simulink subsystem "altitude_controller"  (R2020a)
settings: Solver=VariableStepAuto  StartTime=0.0  StopTime=10.0  RelTol=1e-3
values from neighbouring files (symbols this model uses):
  balloon_fill_mass = max([      gas_for_equilibrium_at_target, ... (first row only)    [configure_simulation.m]    (also in test_kalman.m = 1.8812)
  combined_dry_mass = payload_dry_mass+m_balloon    [configure_simulation.m]
  consumable_mass = 0.5    [configure_simulation.m]    (also in test_kalman.m = 1)
  delay_altitude = target_altitude-5000    (= 19000)    [configure_simulation.m]
  delay_time = 500    [configure_simulation.m]
  dt = 0.01    [configure_simulation.m]    (also in test_kalman.m)
  max_deadzone_error = 100    [configure_simulation.m]
  max_deadzone_speed = 0.2    [configure_simulation.m]
  mdot_ballast = 0.010    (= 0.01)    [configure_simulation.m]
  mdot_ballast_noise_power = 0.0001    [configure_simulation.m]
  mdot_bleed = 0.010    (= 0.01)    [configure_simulation.m]
  mdot_bleed_noise_power = 0.0001    [configure_simulation.m]
  min_altitude_limit = 15000    [configure_simulation.m]
  target_altitude = 24000    [configure_simulation.m]    (also in linearization.m)
undefined symbols (not defined in the file or in its folder): Dump, enum_ControlMode, max_safe_error, Vent
libraries: simulink x6
settings Model: Creator=Philip  LastModifiedBy=Philip

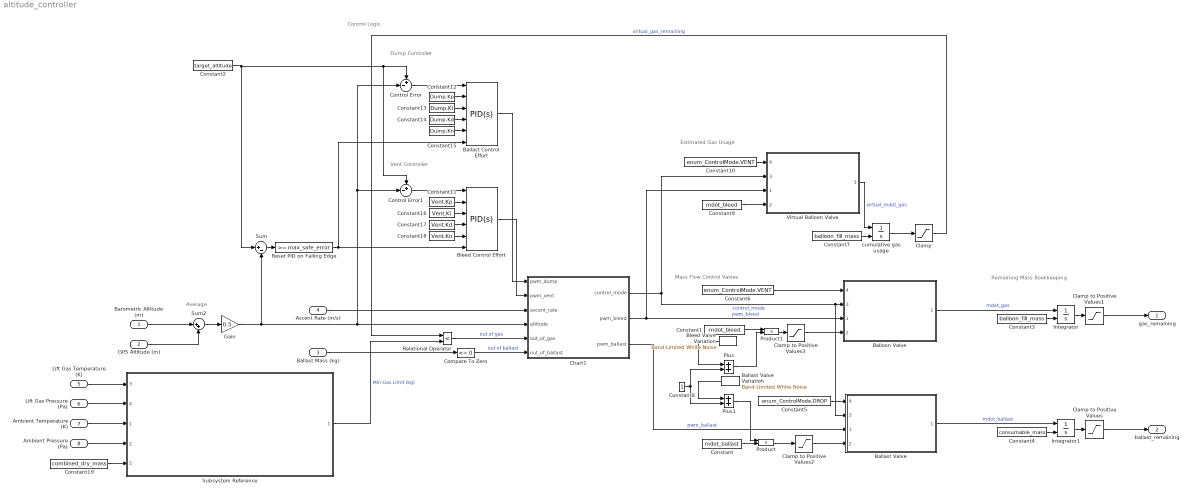
== system altitude_controller ==
  note: Average
  note: Estimated Gas Usage
  note: Remaining Mass Bookkeeping
  note: Mass Flow Control Valves
  note: Control Logic
  note: Dump Controller
  note: Vent Controller
  Barometric Altitude (m) : Inport  Unit=m
  GPS Altitude (m) : Inport  Port=2  OutMin=0  Unit=m
  Ballast Mass (kg) : Inport  Port=3  Unit=kg
  Ascent Rate (m/s) : Inport  Port=4
  Lift Gas Temperature (K) : Inport  Port=5
  Lift Gas Pressure (Pa) : Inport  Port=6
  Ambient Temperature (K) : Inport  Port=7
  Ambient Pressure (Pa) : Inport  Port=8
  Ballast Control Effort : simulink/Continuous/PID Controller  Controller=PID  Form=Parallel  TimeDomain=Continuous-time  UseExternalTs=off  SampleTime=1  IntegratorMethod=Forward Euler  FilterMethod=Forward Euler  ControllerParametersSource=external  P=1  I=1  D=0  UseFilter=on  N=100  TunerSelectOption=Transfer Function Based (PID Tuner App)  InitialConditionSource=internal  InitialConditionForIntegrator=0  InitialConditionForFilter=0  DifferentiatorICPrevScaledInput=0  ExternalReset=falling  TrackingMode=off  Kt=1  LimitOutput=on  UpperSaturationLimit=1  LowerSaturationLimit=0  LinearizeAsGain=on  AntiWindupMode=clamping  Kb=Dump.Kb  POutMin=[]  POutMax=[]  IOutMin=[]  IOutMax=[]  DOutMin=[]  DOutMax=[]  NOutMin=[]  NOutMax=[]  SumOutMin=[]  SumOutMax=[]  SaturationOutMin=[]  SaturationOutMax=[]  PParamMin=[]  PParamMax=[]  IParamMin=[]  IParamMax=[]  DParamMin=[]  DParamMax=[]  NParamMin=[]  NParamMax=[]  KbParamMin=[]  KbParamMax=[]  KtParamMin=[]  KtParamMax=[]  KbOutMin=[]  KbOutMax=[]  KtOutMin=[]  KtOutMax=[]  IntegratorOutMin=[]  IntegratorOutMax=[]  FilterOutMin=[]  FilterOutMax=[]  SumI1OutMin=[]  SumI1OutMax=[]  SumI2OutMin=[]  SumI2OutMax=[]  SumI3OutMin=[]  SumI3OutMax=[]  SumI4OutMin=[]  SumI4OutMax=[]  SumDOutMin=[]  SumDOutMax=[]  DifferentiatorOutMin=[]  DifferentiatorOutMax=[]  FilterDiffOutCoefMin=[]  FilterDiffOutCoefMax=[]  ReciprocalOutMin=[]  ReciprocalOutMax=[]  SumDenOutMin=[]  SumDenOutMax=[]  SumNumOutMin=[]  SumNumOutMax=[]  DivideOutMin=[]  DivideOutMax=[]  UdiffTsProdOutMin=[]  UdiffTsProdOutMax=[]  NTsProdOutMin=[]  NTsProdOutMax=[]  UintegralTsProdOutMin=[]  UintegralTsProdOutMax=[]  UngainTsProdOutMin=[]  UngainTsProdOutMax=[]  IntegratorContinuousStateAttributes=''  IntegratorStateMustResolveToSignalObject=off  IntegratorRTWStateStorageClass=Auto  FilterContinuousStateAttributes=''  FilterStateMustResolveToSignalObject=off  FilterRTWStateStorageClass=Auto  ParallelPVariant=ExternalParameters  IdealPVariant=Disabled  IVariant=ExternalParameters  DVariant=ExternalParameters  IntegratorVariant=Continuous  SatVariant=Enabled  AWVariant=ContClampingParallel  PCopyVariant=Disabled  TRVariant=Disabled  FdbkBlocksVariant=Forward  IdealPFdbkVariant=Disabled  SatFdbkVariant=Disabled  DerivativeFilterVariant=ContFilter  NVariant=ExternalParameters  NCopyVariant=Disabled  FilterICVariant=InternalICsFilter  IntegratorICVariant=InternalICs  ExternalResetVariant=ExternalReset  TRSumVariant=Passthrough  SumFdbkVariant=Disabled  SumVariant=Sum_PID  TsampFilterVariant=InternalTs  TsampNgainVariant=Passthrough  TsampIntegralVariant=Passthrough
  Ballast Valve : Subsystem  ReferencedSubsystem=valve
      settings: PortSchema="{\"entries\":[{\"content\":{\"sides\":[{\"content\":{\"connectorIds\":[\"In4\",\"In3\",\"In1\",\"In2\"]},\"type\":\"ConnectorPlacement.EquallySpacedRectSide\",\"uuid\":\"d5a4010a-716b-4c41-b50e-e3f8d41c00fa\"},{\"content\":{\"connectorIds\":[\"Out1\"],\"side\":\"RIGHT\"},\"type\":\"ConnectorPlacement.EquallySpacedRectSide\",\"uuid\":\"84ee04a9-1f76-49d4-8ce5-74c0c61315ea\"},{\"content\":{\"connectorIds\":[],\"side\":\"TOP\"},\"type\":\"ConnectorPlacement.EquallySpacedRectSide\",\"uuid\":\"9a241f2e-f8fa-498b-86e9-62cebb811964\"}]},\"type\":\"ConnectorPlacement.EquallySpacedConnector\",\"uuid\":\"72a58c4e-cce1-459e-8fb4-8117f4ed8ad0\"}],\"packageUris\":[\"http://schema.mathworks.com/mf0/Connector/19700101\"],\"version\":\"1.0\"}"
  Ballast Valve Variation : simulink/Sources/Band-Limited White Noise  Cov=[mdot_ballast_noise_power]  Ts=dt  seed=[99]
  Balloon Valve : Subsystem  ReferencedSubsystem=valve
      settings: PortSchema="{\"entries\":[{\"content\":{\"sides\":[{\"content\":{\"connectorIds\":[\"In4\",\"In3\",\"In1\",\"In2\"]},\"type\":\"ConnectorPlacement.EquallySpacedRectSide\",\"uuid\":\"cdbf3294-d966-4e16-a090-5ac559dd01c8\"},{\"content\":{\"connectorIds\":[\"Out1\"],\"side\":\"RIGHT\"},\"type\":\"ConnectorPlacement.EquallySpacedRectSide\",\"uuid\":\"4c7f19d8-188a-43e8-a047-f5757586a2e9\"},{\"content\":{\"connectorIds\":[],\"side\":\"TOP\"},\"type\":\"ConnectorPlacement.EquallySpacedRectSide\",\"uuid\":\"2716a85f-c06c-41ed-9767-e4fda0675730\"}]},\"type\":\"ConnectorPlacement.EquallySpacedConnector\",\"uuid\":\"d3907e4d-f270-4849-a389-21fc81be0f9b\"}],\"packageUris\":[\"http://schema.mathworks.com/mf0/Connector/19700101\"],\"version\":\"1.0\"}"
  Bleed Control Effort : simulink/Continuous/PID Controller  Controller=PID  Form=Parallel  TimeDomain=Continuous-time  UseExternalTs=off  SampleTime=1  IntegratorMethod=Forward Euler  FilterMethod=Forward Euler  ControllerParametersSource=external  P=1  I=1  D=0  UseFilter=on  N=100  TunerSelectOption=Transfer Function Based (PID Tuner App)  InitialConditionSource=internal  InitialConditionForIntegrator=0  InitialConditionForFilter=0  DifferentiatorICPrevScaledInput=0  ExternalReset=falling  TrackingMode=off  Kt=1  LimitOutput=on  UpperSaturationLimit=0  LowerSaturationLimit=-1  LinearizeAsGain=on  AntiWindupMode=clamping  Kb=Vent.Kb  POutMin=[]  POutMax=[]  IOutMin=[]  IOutMax=[]  DOutMin=[]  DOutMax=[]  NOutMin=[]  NOutMax=[]  SumOutMin=[]  SumOutMax=[]  SaturationOutMin=[]  SaturationOutMax=[]  PParamMin=[]  PParamMax=[]  IParamMin=[]  IParamMax=[]  DParamMin=[]  DParamMax=[]  NParamMin=[]  NParamMax=[]  KbParamMin=[]  KbParamMax=[]  KtParamMin=[]  KtParamMax=[]  KbOutMin=[]  KbOutMax=[]  KtOutMin=[]  KtOutMax=[]  IntegratorOutMin=[]  IntegratorOutMax=[]  FilterOutMin=[]  FilterOutMax=[]  SumI1OutMin=[]  SumI1OutMax=[]  SumI2OutMin=[]  SumI2OutMax=[]  SumI3OutMin=[]  SumI3OutMax=[]  SumI4OutMin=[]  SumI4OutMax=[]  SumDOutMin=[]  SumDOutMax=[]  DifferentiatorOutMin=[]  DifferentiatorOutMax=[]  FilterDiffOutCoefMin=[]  FilterDiffOutCoefMax=[]  ReciprocalOutMin=[]  ReciprocalOutMax=[]  SumDenOutMin=[]  SumDenOutMax=[]  SumNumOutMin=[]  SumNumOutMax=[]  DivideOutMin=[]  DivideOutMax=[]  UdiffTsProdOutMin=[]  UdiffTsProdOutMax=[]  NTsProdOutMin=[]  NTsProdOutMax=[]  UintegralTsProdOutMin=[]  UintegralTsProdOutMax=[]  UngainTsProdOutMin=[]  UngainTsProdOutMax=[]  IntegratorContinuousStateAttributes=''  IntegratorStateMustResolveToSignalObject=off  IntegratorRTWStateStorageClass=Auto  FilterContinuousStateAttributes=''  FilterStateMustResolveToSignalObject=off  FilterRTWStateStorageClass=Auto  ParallelPVariant=ExternalParameters  IdealPVariant=Disabled  IVariant=ExternalParameters  DVariant=ExternalParameters  IntegratorVariant=Continuous  SatVariant=Enabled  AWVariant=ContClampingParallel  PCopyVariant=Disabled  TRVariant=Disabled  FdbkBlocksVariant=Forward  IdealPFdbkVariant=Disabled  SatFdbkVariant=Disabled  DerivativeFilterVariant=ContFilter  NVariant=ExternalParameters  NCopyVariant=Disabled  FilterICVariant=InternalICsFilter  IntegratorICVariant=InternalICs  ExternalResetVariant=ExternalReset  TRSumVariant=Passthrough  SumFdbkVariant=Disabled  SumVariant=Sum_PID  TsampFilterVariant=InternalTs  TsampNgainVariant=Passthrough  TsampIntegralVariant=Passthrough
  Bleed Valve Variation : simulink/Sources/Band-Limited White Noise  Cov=[mdot_bleed_noise_power]  Ts=dt  seed=[54321]
  Chart1 : Stateflow chart  TreatAsAtomicUnit=on
      settings: PortSchema="{\"entries\":[{\"content\":{\"sides\":[{\"content\":{\"connectorIds\":[\"In4\",\"In5\",\"In6\",\"In1\",\"In3\",\"In2\"]},\"type\":\"ConnectorPlacement.EquallySpacedRectSide\",\"uuid\":\"64d63616-449e-43a6-adda-d3455e6a4541\"},{\"content\":{\"connectorIds\":[\"Out1\",\"Out2\",\"Out3\"],\"side\":\"RIGHT\"},\"type\":\"ConnectorPlacement.EquallySpacedRectSide\",\"uuid\":\"be766ef1-a3f2-4a03-9521-e781b844e2ed\"},{\"content\":{\"connectorIds\":[],\"side\":\"TOP\"},\"type\":\"ConnectorPlacement.EquallySpacedRectSide\",\"uuid\":\"9efceef1-fb0a-45de-a0f9-df77a6037a92\"}]},\"type\":\"ConnectorPlacement.EquallySpacedConnector\",\"uuid\":\"d98ff2da-f1b8-4466-87f6-556c02f19842\"}],\"packageUris\":[\"http://schema.mathworks.com/mf0/Connector/19700101\"],\"version\":\"1.0\"}"
  Clamp : Saturate  UpperLimit=inf  LowerLimit=0
  Clamp to Positive Values{,1..3} (4 alike) : Saturate  UpperLimit=inf  LowerLimit=0
  Compare To Zero : simulink/Logic and Bit Operations/Compare To Zero  relop=<=  OutDataTypeStr=boolean
  Constant : Constant  Value=mdot_ballast
  Constant1 : Constant  Value=mdot_bleed
  Constant10 : Constant  Value=enum_ControlMode.VENT  OutDataTypeStr=Enum: enum_ControlMode
  Constant11 : Constant  Value=Vent.Kp
  Constant12 : Constant  Value=Dump.Kp
  Constant13 : Constant  Value=Dump.Ki
  Constant14 : Constant  Value=Dump.Kd
  Constant15 : Constant  Value=Dump.Kn
  Constant16 : Constant  Value=Vent.Ki
  Constant17 : Constant  Value=Vent.Kd
  Constant18 : Constant  Value=Vent.Kn
  Constant19 : Constant  Value=combined_dry_mass
  Constant2 : Constant  Value=target_altitude
  Constant3 : Constant  Value=balloon_fill_mass
  Constant4 : Constant  Value=consumable_mass
  Constant5 : Constant  Value=enum_ControlMode.DROP  OutDataTypeStr=Enum: enum_ControlMode
  Constant6 : Constant  Value=enum_ControlMode.VENT  OutDataTypeStr=Enum: enum_ControlMode
  Constant7 : Constant  Value=balloon_fill_mass
  Constant8 : Constant
  Constant9 : Constant  Value=mdot_bleed
  Control Error : Sum  Inputs=+-|
  Control Error1 : Sum  Inputs=+-|
  Gain : Gain  Gain=0.5
  Integrator : Integrator  InitialConditionSource=external
  Integrator1 : Integrator  InitialConditionSource=external
  Plus : Sum
  Plus1 : Sum
  Product : Product
  Product1 : Product
  Relational Operator : RelationalOperator  Operator=<  OutDataTypeStr=boolean  RndMeth=Simplest
  Reset PID on Falling Edge : simulink/Logic and Bit Operations/Compare To Constant  relop=>=  const=max_safe_error  OutDataTypeStr=boolean
  Subsystem Reference : Subsystem  ReferencedSubsystem=lift_gas_required_equilibrium
      settings: PortSchema="{\"entries\":[{\"content\":{\"sides\":[{\"content\":{\"connectorIds\":[\"In3\",\"In4\",\"In1\",\"In2\",\"In5\"]},\"type\":\"ConnectorPlacement.EquallySpacedRectSide\",\"uuid\":\"97e3d6d2-28c2-42e6-b964-39b27142bc91\"},{\"content\":{\"connectorIds\":[\"Out1\"],\"side\":\"RIGHT\"},\"type\":\"ConnectorPlacement.EquallySpacedRectSide\",\"uuid\":\"b9c12e6e-d256-428b-98c3-3c91aa5e80c8\"},{\"content\":{\"connectorIds\":[],\"side\":\"TOP\"},\"type\":\"ConnectorPlacement.EquallySpacedRectSide\",\"uuid\":\"e5619dd6-5925-4f6b-8007-455d17ee4107\"}]},\"type\":\"ConnectorPlacement.EquallySpacedConnector\",\"uuid\":\"b8b94ccc-5761-4d17-be3e-38785c31387a\"}],\"packageUris\":[\"http://schema.mathworks.com/mf0/Connector/19700101\"],\"version\":\"1.0\"}"
  Sum : Sum  Inputs=|+-
  Sum2 : Sum  Inputs=|++
  Virtual Balloon Valve : Subsystem  ReferencedSubsystem=valve
      settings: PortSchema="{\"entries\":[{\"content\":{\"sides\":[{\"content\":{\"connectorIds\":[\"In4\",\"In3\",\"In1\",\"In2\"]},\"type\":\"ConnectorPlacement.EquallySpacedRectSide\",\"uuid\":\"cdbf3294-d966-4e16-a090-5ac559dd01c8\"},{\"content\":{\"connectorIds\":[\"Out1\"],\"side\":\"RIGHT\"},\"type\":\"ConnectorPlacement.EquallySpacedRectSide\",\"uuid\":\"4c7f19d8-188a-43e8-a047-f5757586a2e9\"},{\"content\":{\"connectorIds\":[],\"side\":\"TOP\"},\"type\":\"ConnectorPlacement.EquallySpacedRectSide\",\"uuid\":\"2716a85f-c06c-41ed-9767-e4fda0675730\"}]},\"type\":\"ConnectorPlacement.EquallySpacedConnector\",\"uuid\":\"d3907e4d-f270-4849-a389-21fc81be0f9b\"}],\"packageUris\":[\"http://schema.mathworks.com/mf0/Connector/19700101\"],\"version\":\"1.0\"}"
  cumulative gas usage : Integrator  InitialConditionSource=external
  gas_remaining : Outport  OutMin=0  Unit=kg
  ballast_remaining : Outport  Port=2  OutMin=0  Unit=kg
  wires:
  Compare To Zero/1 -> Chart1/2(out_of_ballast)  "out of ballast"
  Relational Operator/1 -> Chart1/3(out_of_gas)  "out of gas"
  Chart1/3(pwm_ballast) -> Ballast Valve/1  "pwm_ballast"
  Ballast Control Effort/1 -> Chart1/4(pwm_dump)
  Constant1/1 -> Product1/1
  Integrator/1 -> Clamp to Positive Values1/1
  Balloon Valve/1 -> Integrator/1  "mdot_gas"
  Integrator1/1 -> Clamp to Positive Values/1
  Ballast Valve/1 -> Integrator1/1  "mdot_ballast"
  Constant3/1 -> Integrator/2
  Constant4/1 -> Integrator1/2
  Constant5/1 -> Ballast Valve/4
  Constant6/1 -> Balloon Valve/4
  Clamp to Positive Values/1 -> ballast_remaining/1
  Clamp to Positive Values1/1 -> gas_remaining/1
  Barometric Altitude (m)/1 -> Sum2/1
  Ballast Mass (kg)/1 -> Compare To Zero/1
  Gain/1 -> Sum/2, Chart1/1(altitude), Control Error/2, Control Error1/2
  Constant7/1 -> cumulative gas usage/2
  cumulative gas usage/1 -> Clamp/1
  Chart1/1(control_mode) -> Balloon Valve/3, Ballast Valve/3, Virtual Balloon Valve/3  "control_mode"
  Constant10/1 -> Virtual Balloon Valve/4
  Constant9/1 -> Virtual Balloon Valve/2
  Chart1/2(pwm_bleed) -> Balloon Valve/1, Virtual Balloon Valve/1  "pwm_bleed"
  Virtual Balloon Valve/1 -> cumulative gas usage/1  "virtual_mdot_gas"
  Clamp/1 -> Relational Operator/1  "virtual_gas_remaining"
  Product1/1 -> Clamp to Positive Values3/1
  Product/1 -> Clamp to Positive Values2/1
  Sum2/1 -> Gain/1
  Clamp to Positive Values2/1 -> Ballast Valve/2
  Clamp to Positive Values3/1 -> Balloon Valve/2
  Bleed Valve Variation/1 -> Plus/1
  Plus/1 -> Product1/2
  Constant8/1 -> Plus/2, Plus1/2
  Ballast Valve Variation/1 -> Plus1/1
  Constant/1 -> Product/2
  Plus1/1 -> Product/1
  Bleed Control Effort/1 -> Chart1/5(pwm_vent)
  Constant13/1 -> Ballast Control Effort/3
  Constant12/1 -> Ballast Control Effort/2
  Constant14/1 -> Ballast Control Effort/4
  Constant15/1 -> Ballast Control Effort/5
  Constant2/1 -> Control Error/1, Control Error1/1, Sum/1
  Control Error1/1 -> Bleed Control Effort/1
  Constant11/1 -> Bleed Control Effort/2
  Constant16/1 -> Bleed Control Effort/3
  Constant17/1 -> Bleed Control Effort/4
  Constant18/1 -> Bleed Control Effort/5
  Ascent Rate (m/s)/1 -> Chart1/6(ascent_rate)
  Reset PID on Falling Edge/1 -> Ballast Control Effort/6, Bleed Control Effort/6
  Sum/1 -> Reset PID on Falling Edge/1
  Control Error/1 -> Ballast Control Effort/1
  GPS Altitude (m)/1 -> Sum2/2
  Lift Gas Temperature (K)/1 -> Subsystem Reference/3
  Lift Gas Pressure (Pa)/1 -> Subsystem Reference/4
  Ambient Pressure (Pa)/1 -> Subsystem Reference/2
  Ambient Temperature (K)/1 -> Subsystem Reference/1
  Subsystem Reference/1 -> Relational Operator/2  "Min Gas Limit (kg)"
  Constant19/1 -> Subsystem Reference/5

== stateflow chart altitude_controller/Chart1 ==
  state Armed
    state Cruise
      control_mode = IDLE;
      pwm_bleed = 0;
      pwm_ballast = 0;
      settings: description=The manifold pressure sensor gives a reliable indication of absolute pressure (MAP).
    state Stabilize
      settings: description=The pressure sensor (manifold, or MAP) no longer produces reliable data.
      (history)
      state Idle
        control_mode = IDLE;
        pwm_bleed = 0;
        pwm_ballast = 0;
      state Lower
        control_mode = VENT;
        pwm_bleed = abs(pwm_vent);
        pwm_ballast = 0;
      state Raise
        control_mode = DROP;
        pwm_bleed = 0;
        pwm_ballast = abs(pwm_dump);
      (default) -> Idle
      Idle -> Raise [order 1] : [ascent_rate < 0 & ~out_of_ballast]
      Idle -> Lower [order 2] : [ascent_rate > 0 & ~out_of_gas]
      Raise -> Idle : [ascent_rate >= 0 | out_of_ballast]
      Lower -> Idle : [ascent_rate <= 0 | out_of_gas]
    Stabilize -> Cruise : [abs(target_altitude - altitude) < max_deadzone_error ...
        | & abs(ascent_rate) < max_deadzone_speed]
    Cruise -> Stabilize : [abs(target_altitude - altitude) > max_deadzone_error ...
        | | abs(ascent_rate) > max_deadzone_speed]
  state Disarmed
    state Init
      control_mode = SAFE;
      pwm_bleed = 0;
      pwm_ballast = 0;
    state Safe
      control_mode = SAFE;
      pwm_bleed = 0;
      pwm_ballast = 0;
    state Dump
      control_mode = DROP;
      pwm_bleed = 0;
      pwm_ballast = 1;
    Dump -> Safe : [out_of_ballast]
  (default) -> Init
  Init -> Stabilize : [after(delay_time,sec) & altitude > delay_altitude]
  Armed -> Safe [order 1] : [out_of_ballast & out_of_gas]
  Armed -> Dump [order 2] : [altitude < min_altitude_limit]
  data: target_altitude parameter double; control_mode output Enum: enum_ControlMode; altitude input double; out_of_ballast input boolean; out_of_gas input boolean; pwm_bleed output =0; pwm_ballast output =0; delay_altitude parameter; min_altitude_limit parameter; max_deadzone_error parameter; delay_time parameter; pwm_dump input; pwm_vent input; ascent_rate input; max_deadzone_speed parameter
